simulink model "dobby"  (R2017b)
settings: Solver=VariableStepAuto  StartTime=0.0  StopTime=4  RelTol=1e-3
settings Model: Creator=dhruvlaad  LastModifiedBy=dhruvlaad

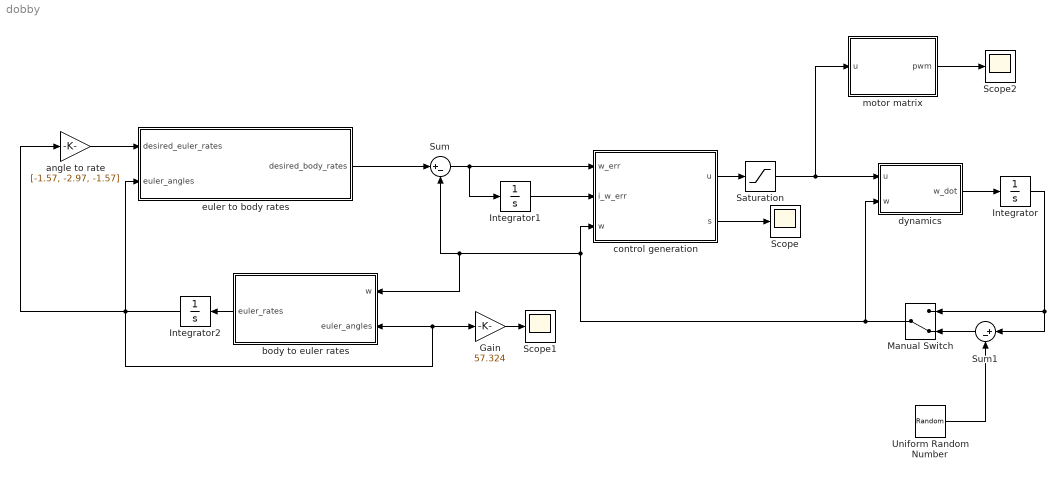
== system dobby ==
  Gain : Gain  Gain=57.324
  Integrator : Integrator  InitialCondition=[0, 0, 0]
  Integrator1 : Integrator  LimitOutput=on  UpperSaturationLimit=[6, 6, 6]  LowerSaturationLimit=[-6, -6, -6]
  Integrator2 : Integrator  InitialCondition=[0, 30*0.0174, 0]
  Manual Switch : ManualSwitch  CurrentSetting=0
  Saturation : Saturate  UpperLimit=64*2  LowerLimit=-64*2
  Scope : Scope
  Scope1 : Scope
  Scope2 : Scope
  Sum : Sum  Inputs=|+-
  Sum1 : Sum  Inputs=|+-
  Uniform Random Number : UniformRandomNumber  Minimum=-0.2  Maximum=0.2  SampleTime=0.01
  angle to rate : Gain  Gain=[-1.57, -2.97, -1.57]
  body to euler rates : MATLAB Function  TreatAsAtomicUnit=on
  control generation : MATLAB Function  TreatAsAtomicUnit=on
  dynamics : MATLAB Function  TreatAsAtomicUnit=on
  "euler to body rates " : MATLAB Function  TreatAsAtomicUnit=on
  motor matrix : MATLAB Function  TreatAsAtomicUnit=on
  wires:
  control generation/1(u) -> Saturation/1
  dynamics/1(w_dot) -> Integrator/1
  "euler to body rates "/1(desired_body_rates) -> Sum/1
  Sum/1 -> Integrator1/1, control generation/1(w_err)
  Integrator1/1 -> control generation/2(i_w_err)
  control generation/2(s) -> Scope/1
  body to euler rates/1(euler_rates) -> Integrator2/1
  Integrator2/1 -> angle to rate/1, Gain/1, body to euler rates/2(euler_angles), "euler to body rates "/2(euler_angles)
  angle to rate/1 -> "euler to body rates "/1(desired_euler_rates)
  Gain/1 -> Scope1/1
  Saturation/1 -> motor matrix/1(u), dynamics/1(u)
  Integrator/1 -> Manual Switch/1, Sum1/1
  Uniform Random Number/1 -> Sum1/2
  Sum1/1 -> Manual Switch/2
  Manual Switch/1 -> body to euler rates/1(w), Sum/2, control generation/3(w), dynamics/2(w)
  motor matrix/1(pwm) -> Scope2/1

== matlab function dobby/control generation ==
  data: w_err input; i_w_err input; w input; u output; s output
function [u, s]= fcn(w_err, i_w_err, w)

Ixx = 1000*(0.000081599 + 0.00032233 + 0.0133609 + 0.0044966);
Iyy = 1000*(0.000586590 + 0.00032233 + 0.0133609 + 0.0044966);
Izz = 1000*(0.000621150 + 0.00032968 + 0.0163521 + 0.0118809);

l1 = 0.0
l2 = 1.98
l3 = 0.0
eta1 = 0.0
eta2 = 0.4
eta3 = 0.0

w_err_1 = w_err(1);
w_err_2 = w_err(2);
w_err_3 = w_err(3);
i_w_err_1 = i_w_err(1);
i_w_err_2 = i_w_err(2);
i_w_err_3 = i_w_err(3);
w1 = w(1);
w2 = w(2);
w3 = w(3);

s1 = w_err_1 + l1*i_w_err_1;
s2 = w_err_2 + l2*i_w_err_2;
s3 = w_err_3 + l3*i_w_err_3;

u1 = (Izz - Iyy)*w2*w3 + Ixx*l1*w_err_1 + eta1*atan(s1);
u2 = (Ixx - Izz)*w1*w3 + Iyy*l2*w_err_2 + eta2*atan(s2);
u3 = (Iyy - Ixx)*w2*w1 + Izz*l3*w_err_3 + eta3*atan(s3);

u = [u1, u2, u3];
s = [s1, s2, s3];

== matlab function dobby/euler to body rates  ==
  data: desired_euler_rates input; desired_body_rates output; euler_angles input
function desired_body_rates = fcn(desired_euler_rates, euler_angles)

phi = euler_angles(1);
theta = euler_angles(2);
psi = euler_angles(3);
phi_dot = desired_euler_rates(1);
theta_dot = desired_euler_rates(2);
psi_dot = desired_euler_rates(3);

w1 = phi_dot - sin(theta)*psi_dot;
w2 = theta_dot*cos(phi) + sin(phi)*cos(theta)*psi_dot;
w3 = cos(phi)*cos(theta)*psi_dot - sin(phi)*theta_dot;

desired_body_rates = [w1, w2, w3]

== matlab function dobby/dynamics ==
  data: u input; w_dot output; w input
function w_dot = fcn(u, w)

Ixx = 1000*(0.000081599 + 0.00032233 + 0.0133609 + 0.0044966);
Iyy = 1000*(0.000586590 + 0.00032233 + 0.0133609 + 0.0044966);
Izz = 1000*(0.000621150 + 0.00032968 + 0.0163521 + 0.0118809);

u1 = u(1);
u2 = u(2);
u3 = u(3);
w1 = w(1);
w2 = w(2);
w3 = w(3);

w1_dot = ((Iyy - Izz)*w2*w3 + u1)/Ixx;
w2_dot = ((Izz - Ixx)*w3*w1 + u2)/Iyy;
w3_dot = ((Ixx - Iyy)*w1*w2 + u3)/Izz;

w_dot = [w1_dot, w2_dot, w3_dot]

== matlab function dobby/body to euler rates ==
  data: w input; euler_rates output; euler_angles input
function euler_rates = fcn(w, euler_angles)

phi = euler_angles(1);
theta = euler_angles(2);
psi = euler_angles(3);
w1 = w(1);
w2 = w(2);
w3 = w(3);

phi_dot = w1 + sin(phi)*tan(theta)*w2 + cos(phi)*tan(theta)*w3;
theta_dot = cos(phi)*w2 - sin(phi)*w3;
psi_dot = (sin(phi)/cos(theta))*w2 + (cos(phi)/cos(theta))*w3;

euler_rates = [phi_dot, theta_dot, psi_dot]

== matlab function dobby/motor matrix ==
  data: u input; pwm output
function pwm = fcn(u)

THRUST_CONST = 967;
MOM_COEFF = 5.917;
THRUST_COEFF = 2.724;

mean_thrust = 4.00*(1500 - THRUST_CONST)*0.367;
u1 = u(1);
u2 = u(2);
u3 = u(3);

t1 = (0.25)*(mean_thrust - (u3) - (u1 + u2)*MOM_COEFF);
t2 = (0.25)*(mean_thrust - (u3) + (u1 + u2)*MOM_COEFF);
t3 = (0.25)*(mean_thrust + (u3) + (u1 - u2)*MOM_COEFF);
t4 = (0.25)*(mean_thrust + (u3) - (u1 - u2)*MOM_COEFF);

pwm1 = t1*THRUST_COEFF + THRUST_CONST;
pwm2 = t2*THRUST_COEFF + THRUST_CONST;
pwm3 = t3*THRUST_COEFF + THRUST_CONST;
pwm4 = t4*THRUST_COEFF + THRUST_CONST;

pwm = [pwm1, pwm2, pwm3, pwm4]
